simulink model "RI_RL_V"  (R2013b)
settings: Solver=ode45  StartTime=0.0  StopTime=25*L/R  MaxStep=tau/100  RelTol=1e-3
InitFcn:
  | % Modellparaméterek
  | R = 250e-3;
  | L = 10e-3;
  | Psi_0 = 0.5e-3;
  | 
  | i_0 = 0;
  | theta_0 = 0;
  | 
  | % Rendszerparaméterek
  | K = 1/R;
  | tau = L/R;
libraries: RI_MK x3, simulink x1
settings Model: Creator=Szalay  LastModifiedBy=Szalay

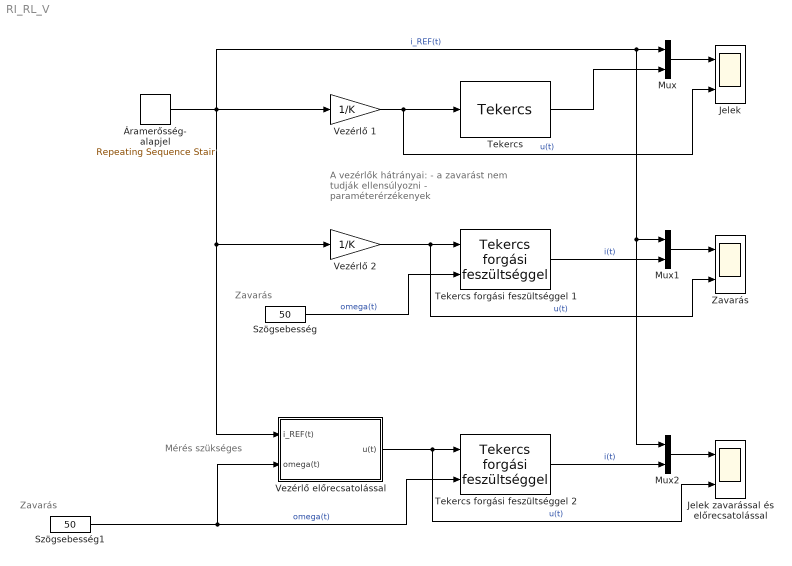
== system RI_RL_V ==
  note: Zavarás
  note: A vezérlők hátrányai:
      | - a zavarást nem tudják ellensúlyozni
      | - paraméterérzékenyek
  note: Zavarás
  note: Mérés
      | szükséges
  Jelek : Scope  NumInputPorts=2
      settings: ShowLegends=on  YMin=-5~-5  YMax=5~5
  Jelek zavarással és előrecsatolással : Scope  NumInputPorts=2
      settings: ShowLegends=on  YMin=-5~-5  YMax=5~5  SaveName=ScopeData2
  Mux : Mux  Inputs=2
  Mux1 : Mux  Inputs=2
  Mux2 : Mux  Inputs=2
  Szögsebesség : Constant  Value=50
  Szögsebesség1 : Constant  Value=50
  Tekercs : RI_MK/Tekercs  R=R  L=L  i_0=0
  Tekercs forgási feszültséggel 1 : RI_MK/Tekercs forgási feszültséggel  R=R  L=L  Psi_0=Psi_0  i_0=i_0  theta_0=theta_0
  Tekercs forgási feszültséggel 2 : RI_MK/Tekercs forgási feszültséggel  R=R  L=L  Psi_0=Psi_0  i_0=i_0  theta_0=theta_0
  Vezérlő 1 : Gain  Gain=1/K
  Vezérlő 2 : Gain  Gain=1/K
  Vezérlő előrecsatolással : Subsystem
  Zavarás : Scope  NumInputPorts=2
      settings: ShowLegends=on  YMin=-5~-5  YMax=5~5
  Áramerősség- alapjel : simulink/Sources/Repeating Sequence Stair  OutValues=[300, 100, -400, 200, -100]*1e-3  tsamp=L/R*5  OutMin=[]  OutMax=[]  OutDataTypeStr=double  OutputDataTypeScalingMode=double  OutDataType=fixdt(0,8)  ConRadixGroup=Best Precision: Vector-wise  OutScaling=2^-12
  wires:
  Mux/1 -> Jelek/1
  Vezérlő 1/1 -> Tekercs/1, Jelek/2  "u(t)"
  Mux1/1 -> Zavarás/1
  Tekercs/1 -> Mux/2
  Szögsebesség/1 -> Tekercs forgási feszültséggel 1/2  "omega(t)"
  Tekercs forgási feszültséggel 1/1 -> Mux1/2  "i(t)"
  Vezérlő 2/1 -> Zavarás/2, Tekercs forgási feszültséggel 1/1  "u(t)"
  Áramerősség- alapjel/1 -> Vezérlő 1/1, Mux2/1, Mux1/1, Mux/1, Vezérlő 2/1, Vezérlő előrecsatolással/1(i_REF(t))  "i_REF(t)"
  Mux2/1 -> Jelek zavarással és előrecsatolással/1
  Szögsebesség1/1 -> Tekercs forgási feszültséggel 2/2, Vezérlő előrecsatolással/2(omega(t))  "omega(t)"
  Tekercs forgási feszültséggel 2/1 -> Mux2/2  "i(t)"
  Vezérlő előrecsatolással/1(u(t)) -> Tekercs forgási feszültséggel 2/1, Jelek zavarással és előrecsatolással/2  "u(t)"

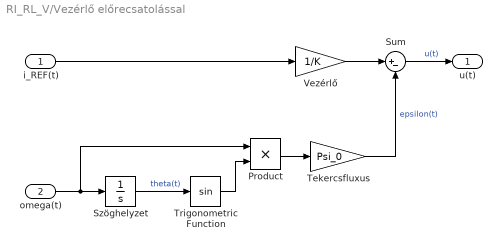
== system RI_RL_V/Vezérlő előrecsatolással ==
  i_REF(t) : Inport
  omega(t) : Inport  Port=2
  Product : Product
  Sum : Sum  Inputs=|+-
  Szöghelyzet : Integrator  InitialCondition=theta_0
  Tekercsfluxus : Gain  Gain=Psi_0
  Trigonometric Function : Trigonometry
  Vezérlő : Gain  Gain=1/K
  u(t) : Outport
  wires:
  Vezérlő/1 -> Sum/1
  Sum/1 -> u(t)/1  "u(t)"
  Szöghelyzet/1 -> Trigonometric Function/1  "theta(t)"
  Trigonometric Function/1 -> Product/2
  Product/1 -> Tekercsfluxus/1
  Tekercsfluxus/1 -> Sum/2  "epsilon(t)"
  omega(t)/1 -> Szöghelyzet/1, Product/1
  i_REF(t)/1 -> Vezérlő/1
